simulink model "LinLongNormal_Aquila_Claws_Discrete"  (Simulink 8.9)
settings: Solver=VariableStepAuto  StartTime=0.0  StopTime=500  RelTol=1e-3  EnableMultiTasking=on
PreLoadFcn:
  | AquilaDiscreteClawsParameters
  | AquilaDiscreteModelParameters
model workspace: external: MAT-File /Users/hbolandhemmat/Dropbox (Facebook)/Aquila/GNC/0_Personal_Folders/Hamidreza Bolandhemmat/Matlab_Projects/Aquila_Claws_Design_Cascaded/utilities/AquilaDiscreteClawsParameters.mat (data not in the file)
undefined symbols (not defined in the file): AP_AltLoop_AltCmdLPFDenTau, AP_AltLoop_Kd, AP_AltLoop_Ki, AP_AltLoop_Ki_WindupMaxLim, AP_AltLoop_Ki_WindupMinLim, AP_AltLoop_Kp, AP_ClimbRate_LPFDenTau, AP_ClimbRateLoop_ClimbRateCmdLPFDenTau, AP_ClimbRateLoop_Ki, AP_ClimbRateLoop_Kp, AP_ClimbRateLoop_LLFiltDenCoe, AP_ClimbRateLoop_LLFiltNumCoe, AP_ClimbRateLoop_MaxPitchCmdrad, AP_ClimbRateLoop_MinPitchCmdrad, AP_GndTrkLoop_CmdLPFDenTau, AP_GndTrkLoop_Kd, AP_GndTrkLoop_Kp, AP_GndTrkLoop_phiCmdMaxLimDeg, AP_GndTrkLoop_phiCmdMinLimDeg, AP_GndTrkLoop_phiRateCmdMaxLimDps, AP_GndTrkLoop_phiRateCmdMinLimDps, AP_PitchLoop_DerivLPFDenTau, AP_PitchLoop_Kd, AP_PitchLoop_Kff, AP_PitchLoop_Ki, AP_PitchLoop_Kp, AP_PitchLoop_Kq, AP_PitchLoop_Notch1BWfactor, AP_PitchLoop_Notch1CosFreqNorm, AP_PitchLoop_qFdbkLFLLFiltDenCoe, AP_PitchLoop_qFdbkLFLLFiltNumCoe, AP_PitchLoop_qFdbkLLFiltDenCoe, AP_PitchLoop_qFdbkLLFiltNumCoe, AP_PitchLoop_thetaCmdLPFDenTau, AP_PitchLoop_wn_ElvRollOff, AP_PitchLoop_zeta_ElvRollOff, AP_PwrLoop_ClimbRateCmdLPFDenTau, AP_PwrLoop_Ki, AP_PwrLoop_Kp, AP_PwrLoop_Kvadv, AP_PwrLoop_LLFiltDenCoe, AP_PwrLoop_LLFiltNumCoe, AP_PwrLoop_MaxThrCmdNorm, AP_PwrLoop_MinThrCmdNorm, AP_PwrLoop_wn_ThrRollOff, AP_PwrLoop_zeta_ThrRollOff, AP_RollLoop_ailCmdMaxLim, AP_RollLoop_ailCmdMinLim, AP_RollLoop_AilWindupMaxLim, AP_RollLoop_AilWindupMinLim, AP_RollLoop_Ki, AP_RollLoop_Kp, AP_RollLoop_KrollrateAdv, AP_RollLoop_Notch1BWfactor, AP_RollLoop_Notch1CosFreqNorm, AP_RollLoop_pFdbkLFLLFiltDenCoe, AP_RollLoop_pFdbkLFLLFiltNumCoe, AP_RollLoop_pFdbkLLFiltDenCoe, AP_RollLoop_pFdbkLLFiltNumCoe, AP_RollLoop_phiErrLPFDenTau ... (+41)
libraries: discretizing x16, aerolibconvert2 x12, simulink x10, cstblocks x1
(part 2 of 2)

== system LinLongNormal_Aquila_Claws_Discrete/Longitudinal_Control_Laws/PitchLoop/Subsystem1 ==
  u : Inport
  AP_PitchLoop_qFdbkLFLLFiltDenCoe : Gain  Gain=AP_PitchLoop_qFdbkLFLLFiltDenCoe
  AP_PitchLoop_qFdbkLFLLFiltNumCoe : Gain  Gain=AP_PitchLoop_qFdbkLFLLFiltNumCoe
  Delay : Delay  DelayLength=1  InitialCondition=0  SampleTime=Ts
  Delay1 : Delay  DelayLength=1  InitialCondition=0  SampleTime=Ts
  Sum3 : Sum  Inputs=+|+|-
  y : Outport
  wires:
  AP_PitchLoop_qFdbkLFLLFiltDenCoe/1 -> Sum3/3
  u/1 -> AP_PitchLoop_qFdbkLFLLFiltNumCoe/1, Sum3/1
  Delay1/1 -> AP_PitchLoop_qFdbkLFLLFiltDenCoe/1
  AP_PitchLoop_qFdbkLFLLFiltNumCoe/1 -> Delay/1
  Delay/1 -> Sum3/2
  Sum3/1 -> y/1, Delay1/1

== system LinLongNormal_Aquila_Claws_Discrete/Longitudinal_Control_Laws/PwrLoop/Subsystem ==
  u : Inport
  AP_PwrLoop_LLFiltDenCoe : Gain  Gain=AP_PwrLoop_LLFiltDenCoe
  AP_PwrLoop_LLFiltNumCoe : Gain  Gain=AP_PwrLoop_LLFiltNumCoe
  Delay : Delay  DelayLength=1  InitialCondition=0  SampleTime=Ts
  Delay1 : Delay  DelayLength=1  InitialCondition=0  SampleTime=Ts
  Sum3 : Sum  Inputs=+|+|-
  y : Outport
  wires:
  AP_PwrLoop_LLFiltDenCoe/1 -> Sum3/3
  u/1 -> AP_PwrLoop_LLFiltNumCoe/1, Sum3/1
  Delay1/1 -> AP_PwrLoop_LLFiltDenCoe/1
  AP_PwrLoop_LLFiltNumCoe/1 -> Delay/1
  Delay/1 -> Sum3/2
  Sum3/1 -> y/1, Delay1/1

== system LinLongNormal_Aquila_Claws_Discrete/Longitudinal_Control_Laws/SpeedLoop/Subsystem ==
  u : Inport
  AP_TASLoop_LLFiltDenCoe : Gain  Gain=AP_TASLoop_LLFiltDenCoe
  AP_TASLoop_LLFiltNumCoe : Gain  Gain=AP_TASLoop_LLFiltNumCoe
  Delay : Delay  DelayLength=1  InitialCondition=0  SampleTime=Ts
  Delay1 : Delay  DelayLength=1  InitialCondition=0  SampleTime=Ts
  Sum3 : Sum  Inputs=+|+|-
  y : Outport
  wires:
  AP_TASLoop_LLFiltDenCoe/1 -> Sum3/3
  u/1 -> AP_TASLoop_LLFiltNumCoe/1, Sum3/1
  Delay1/1 -> AP_TASLoop_LLFiltDenCoe/1
  AP_TASLoop_LLFiltNumCoe/1 -> Delay/1
  Delay/1 -> Sum3/2
  Sum3/1 -> y/1, Delay1/1
